simulink model "relu_int"  (R2024b)
settings: Solver=VariableStepAuto  StartTime=0.0  StopTime=10  RelTol=1e-3
InitFcn:
  | % Define a random matrix size between 3 and 10
  | n = randi([3, 10]);
  | 
  | fprintf('Size of matrix A: n = %d\n', n);
settings Model: Creator=valen  LastModifiedBy=valen
settings OptimizationCC: BlockReduction=off  ConditionallyExecuteInputs=off
settings HardwareCC: ProdBitPerPointer=32  ProdBitPerSizeT=32  ProdBitPerPtrDiffT=32  ProdLargestAtomicFloat=None  ProdIntDivRoundTo=Undefined  ProdEndianess=Unspecified  ProdWordSize=32  ProdHWDeviceType=ASIC/FPGA->ASIC/FPGA  TargetBitPerPointer=64  TargetBitPerSizeT=64  TargetBitPerPtrDiffT=64  TargetLongLongMode=on  TargetIntDivRoundTo=Zero  TargetEndianess=LittleEndian  TargetWordSize=64  TargetHWDeviceType=Custom Processor->MATLAB Host Computer  ProdEqTarget=off

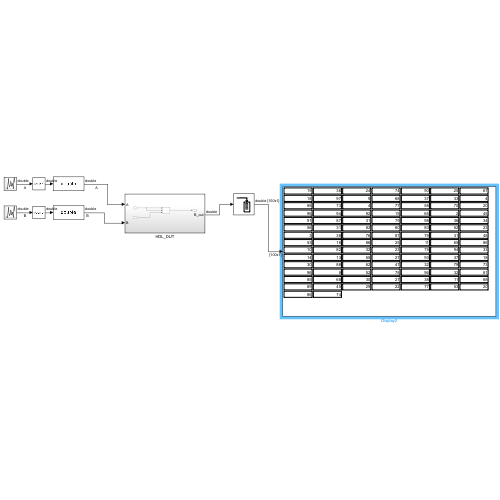
[thumbnail: Simulink's stored preview of the top-level diagram]
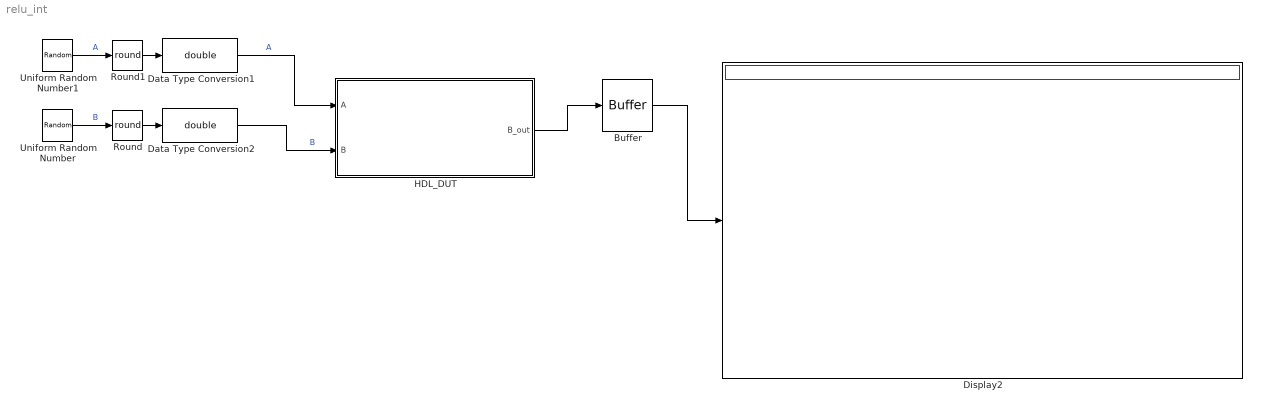
== system relu_int ==
  Buffer : Buffer  N=n*n  OutputFrames=off
  Data Type Conversion1 : DataTypeConversion  OutDataTypeStr=double  SaturateOnIntegerOverflow=off  RndMeth=Floor
  Data Type Conversion2 : DataTypeConversion  OutDataTypeStr=double  SaturateOnIntegerOverflow=off  RndMeth=Floor
  Display2 : Display
  HDL_DUT : Subsystem
  Round : Rounding  Operator=round
  Round1 : Rounding  Operator=round
  Uniform Random Number : UniformRandomNumber  Minimum=0  Maximum=100  Seed=randi([0,100])  SampleTime=10/(n*n)
  Uniform Random Number1 : UniformRandomNumber  Minimum=0  Maximum=100  Seed=randi([0,100])  SampleTime=10/(n*n)
  wires:
  HDL_DUT/1(B_out) -> Buffer/1
  Buffer/1 -> Display2/1
  Data Type Conversion1/1 -> HDL_DUT/1(A)  "A"
  Data Type Conversion2/1 -> HDL_DUT/2(B)  "B"
  Uniform Random Number/1 -> Round/1  "B"
  Round/1 -> Data Type Conversion2/1
  Round1/1 -> Data Type Conversion1/1
  Uniform Random Number1/1 -> Round1/1  "A"

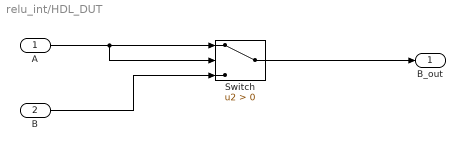
== system relu_int/HDL_DUT ==
  A : Inport
  B : Inport  Port=2
  Switch : Switch  Criteria=u2 > Threshold  SaturateOnIntegerOverflow=off  InputSameDT=off
  B_out : Outport  VectorParamsAs1DForOutWhenUnconnected=off
  wires:
  A/1 -> Switch/2, Switch/1
  B/1 -> Switch/3
  Switch/1 -> B_out/1
